simulink model "sism_integral"  (R2023b)
settings: Solver=FixedStepAuto  StartTime=0.0  StopTime=30  FixedStep=t_step  RelTol=1e-3
settings Model: Creator=afons  LastModifiedBy=afons

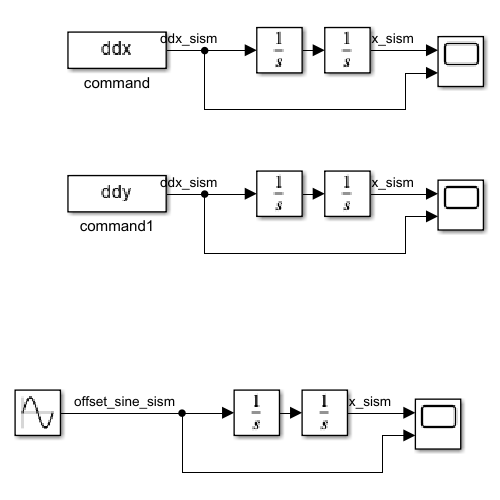
[thumbnail: Simulink's stored preview of the top-level diagram]
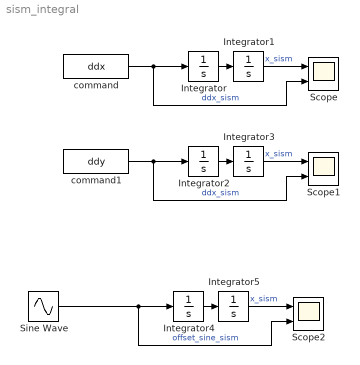
== system sism_integral ==
  Integrator{,1..5} (6 alike) : Integrator
  Scope : Scope  NumInputPorts=2
  Scope1 : Scope  NumInputPorts=2
  Scope2 : Scope  NumInputPorts=2
  Sine Wave : Sin  Bias=0.1  Frequency=20  SampleTime=0
  command : FromWorkspace  VariableName=ddx
  command1 : FromWorkspace  VariableName=ddy
  wires:
  Integrator1/1 -> Scope/1  "x_sism"
  Integrator/1 -> Integrator1/1
  command/1 -> Scope/2, Integrator/1  "ddx_sism"
  command1/1 -> Scope1/2, Integrator2/1  "ddx_sism"
  Integrator2/1 -> Integrator3/1
  Integrator3/1 -> Scope1/1  "x_sism"
  Integrator5/1 -> Scope2/1  "x_sism"
  Integrator4/1 -> Integrator5/1
  Sine Wave/1 -> Scope2/2, Integrator4/1  "offset_sine_sism"
